simulink model "Q1"  (R2018a)
settings: Solver=VariableStepAuto  StartTime=0.0  StopTime=2  RelTol=1e-3
undefined symbols (not defined in the file): a
libraries: powerlib x11, dspstat3 x1, powerlib_meascontrol x1
settings Model: Creator=enes_  LastModifiedBy=enes_

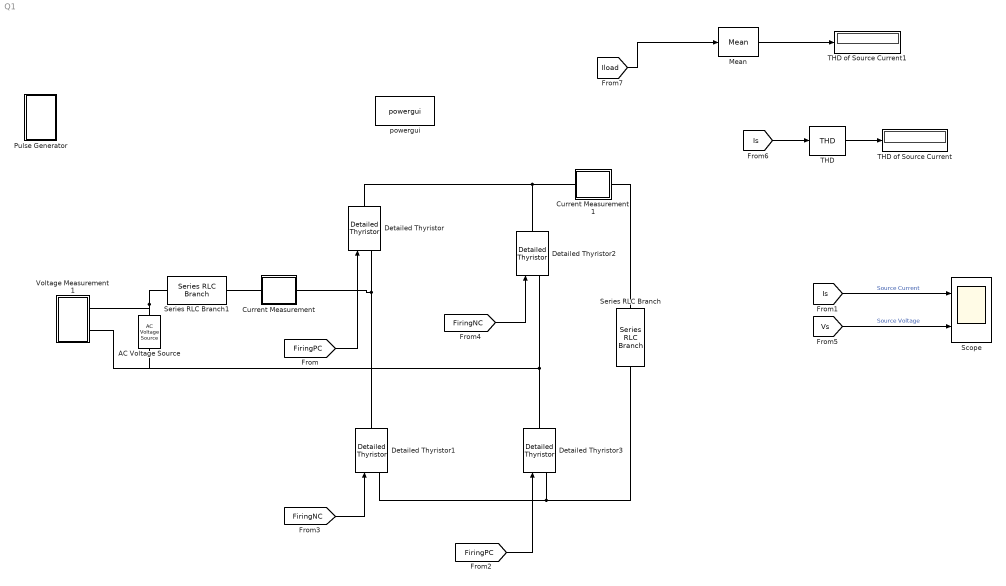
== system Q1 ==
  AC Voltage Source : powerlib/Electrical Sources/AC Voltage Source  Amplitude=326.6  Phase=0  Frequency=50  SampleTime=0  Measurements=None  BusType=swing  Pref=10e3  Qref=0  Qmin=-inf  Qmax=+inf
  Current Measurement : Subsystem
  Current Measurement1 : Subsystem
  Detailed Thyristor{,1..3} (4 alike) : powerlib/Power Electronics/Detailed Thyristor  Ron=0.001  Lon=1e-3  Vf=0.001  IL=0.1  Tq=100e-6  IC=0  Rs=500  Cs=250e-9  Measurements=off
      settings: SourceProductName=Simscape Power Systems  SourceProductBaseCode=PS
  Mean : dspstat3/Mean  run=off  InputProcessing=Columns as channels (frame based)  reset_popup=None  directionMode=Each column  dimension=1  roiEnable=off  roiType=Rectangles  roiPortion=Entire ROI  roiOutput=Individual statistics for each ROI  roiFlag=off  roundingMode=Floor  overflowMode=off  outputDataTypeStr=Inherit: Same as accumulator  outputMin=[]  outputMax=[]  outputLastDataTypeStr=Inherit: Same as accumulator
  Pulse Generator : Subsystem
  Scope : Scope  NumInputPorts=2
  Series RLC Branch : powerlib/Elements/Series RLC Branch  LConnTagsString=__new0  RConnTagsString=__new0  BranchType=RL  Resistance=4  Inductance=200e-3  SetiL0=off  InitialCurrent=0  Capacitance=1e-6  Setx0=off  InitialVoltage=0  Measurements=None
  Series RLC Branch1 : powerlib/Elements/Series RLC Branch  LConnTagsString=__new0  RConnTagsString=__new0  BranchType=L  Resistance=4  Inductance=0.5e-3  SetiL0=off  InitialCurrent=0  Capacitance=1e-6  Setx0=off  InitialVoltage=0  Measurements=None
  THD : powerlib_meascontrol/Measurements/THD  Freq=50  Ts=0
  THD of Source Current : Display
  THD of Source Current1 : Display
  Voltage Measurement1 : Subsystem
  powergui : powerlib/powergui  Priority=1  SimulationMode=Discrete  SampleTime=5e-6  frequency=60  Iterations=50  frequencyindice=50  Pbase=100e6  ErrMax=1e-4  UnitsV=kV  UnitsW=MW  buscounter=0  FunctionMessages=off  echomessages=off  EnableUseOfTLC=off  CurrentSourceSwitches=off  DisableSnubberDevices=off  DisableRonSwitches=off  DisableVfSwitches=off  DisplayEquations=off  SolverType=Tustin/Backward Euler (TBE)  Interpol=off  ExternalGateDelay=off  methode=off  Ts=100  x0status=blocks  SPID=on  SwTol=0  HookPort=off  RestoreLinks=warning  ResistiveCurrentMeasurement=off  Frange=[0:2:500]  Ylog=off  Xlog=on  ShowGrid=off  save=off  variable=ZData  structure=0  ZoomFFT=off  StartTime=0.0  cycles=1  DisplayStyle=1  fundamental=60  FreqAxis=off  MaxFrequency=1000  frequencyindicesteady=1  RmsSteady=1  display=off
  wires:
  [FiringPC] -> Detailed Thyristor/1
  [FiringPC] -> Detailed Thyristor3/1
  [FiringNC] -> Detailed Thyristor1/1
  [FiringNC] -> Detailed Thyristor2/1
  [Is] -> Scope/1  "Source Current"
  [Vs] -> Scope/2  "Source Voltage"
  [Is] -> THD/1
  THD/1 -> THD of Source Current/1
  [Iload] -> Mean/1
  Mean/1 -> THD of Source Current1/1
  connections:
  AC Voltage Source/RConn1 -- Series RLC Branch1/LConn1 -- Voltage Measurement1/LConn1
  Detailed Thyristor3/RConn1 -- Voltage Measurement1/LConn2 -- AC Voltage Source/LConn1 -- Detailed Thyristor2/LConn1
  Detailed Thyristor1/LConn1 -- Series RLC Branch/RConn1 -- Detailed Thyristor3/LConn1
  Detailed Thyristor/RConn1 -- Current Measurement1/LConn1 -- Detailed Thyristor2/RConn1
  Detailed Thyristor1/RConn1 -- Current Measurement/RConn1 -- Detailed Thyristor/LConn1
  Current Measurement/LConn1 -- Series RLC Branch1/RConn1
  Series RLC Branch/LConn1 -- Current Measurement1/RConn1

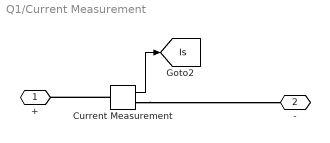
== system Q1/Current Measurement ==
  Current Measurement : powerlib/Measurements/Current Measurement  PhasorSimulation=off  OutputType=Complex  PSBequivalent=0
  + : PMIOPort  Side=Left
  - : PMIOPort  Port=2  Side=Right
  tag scope: Is=global
  wires:
  Current Measurement/1 -> [Is]
  connections:
  Current Measurement/RConn1 -- -/RConn1
  Current Measurement/LConn1 -- +/RConn1

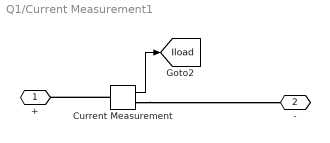
== system Q1/Current Measurement1 ==
  Current Measurement : powerlib/Measurements/Current Measurement  PhasorSimulation=off  OutputType=Complex  PSBequivalent=0
  + : PMIOPort  Side=Left
  - : PMIOPort  Port=2  Side=Right
  tag scope: Iload=global
  wires:
  Current Measurement/1 -> [Iload]
  connections:
  Current Measurement/RConn1 -- -/RConn1
  Current Measurement/LConn1 -- +/RConn1

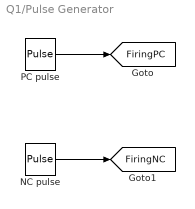
== system Q1/Pulse Generator ==
  NC pulse : DiscretePulseGenerator  PulseType=Time based  Period=1/50  PulseWidth=5  PhaseDelay=a/(100*pi)+1/100
  PC pulse : DiscretePulseGenerator  PulseType=Time based  Period=1/50  PulseWidth=5  PhaseDelay=a/(100*pi)
  tag scope: FiringNC=global, FiringPC=global
  wires:
  PC pulse/1 -> [FiringPC]
  NC pulse/1 -> [FiringNC]

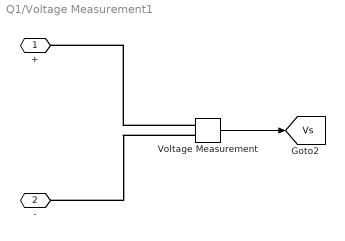
== system Q1/Voltage Measurement1 ==
  Voltage Measurement : powerlib/Measurements/Voltage Measurement  PhasorSimulation=off  OutputType=Complex  PSBequivalent=0
  + : PMIOPort  Side=Left
  - : PMIOPort  Port=2  Side=Left
  tag scope: Vs=global
  wires:
  Voltage Measurement/1 -> [Vs]
  connections:
  Voltage Measurement/LConn2 -- -/RConn1
  Voltage Measurement/LConn1 -- +/RConn1
